simulink subsystem "PieroControladorS"  (R2023b)
settings: Solver=VariableStepAuto  StartTime=0.0  StopTime=10.0  RelTol=1e-3
settings Model: Creator=jaime  LastModifiedBy=jaime

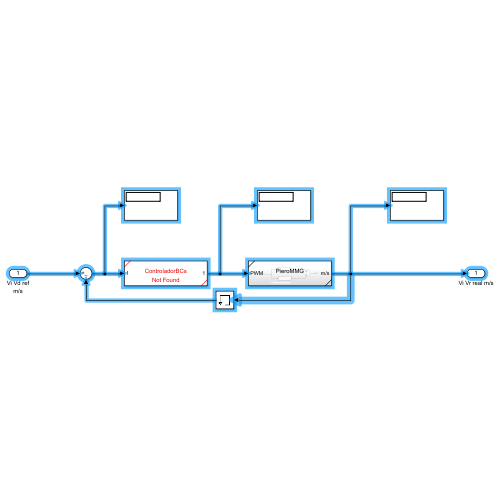
[thumbnail: Simulink's stored preview of the top-level diagram]
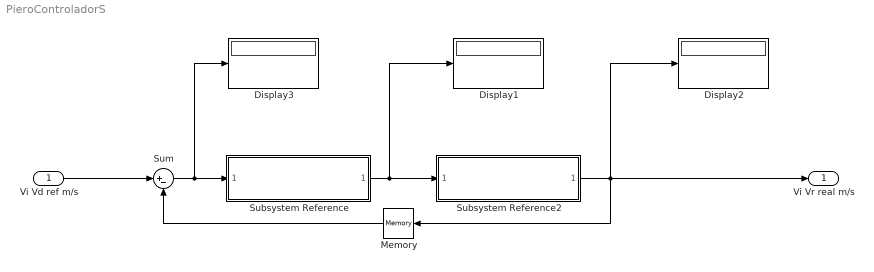
== system PieroControladorS ==
  Vi Vd ref m/s : Inport  OutDataTypeStr=double  PortDimensions=2
  Display1 : Display
  Display2 : Display
  Display3 : Display
  Memory : Memory
  Subsystem Reference : Subsystem  ReferencedSubsystem=ControladorBCs
  Subsystem Reference2 : Subsystem  ReferencedSubsystem=PieroMMG
  Sum : Sum  Inputs=|+-
  Vi Vr real m/s : Outport  OutDataTypeStr=double  PortDimensions=2
  wires:
  Subsystem Reference/1 -> Display1/1, Subsystem Reference2/1
  Memory/1 -> Sum/2
  Sum/1 -> Subsystem Reference/1, Display3/1
  Vi Vd ref m/s/1 -> Sum/1
  Subsystem Reference2/1 -> Memory/1, Vi Vr real m/s/1, Display2/1
